simulink model "DC_DC_buck_Microgrid_sim_1_2_3"  (R2023a)
settings: Solver=ode23tb  StartTime=0.0  StopTime=0.05  MaxStep=1/fpwm/200  RelTol=1e-3  EnableMultiTasking=on
values from neighbouring files (symbols this model uses):
  Cf = 2*IoAVmin/(8*fpwm*DeltaVo*Vo)    (= 5.42534722222e-05)    [DC_DC_buck_Microgrid_1_2_3.m]    (also in DC_DC_buck_Microgrid_4.m = 2.71267361111e-05)
  deltaN = Vo/U    (= 0.48)    [DC_DC_buck_Microgrid_1_2_3.m]    (also in DC_DC_buck_Microgrid_4.m)
  fpwm = 10000    [DC_DC_buck_Microgrid_1_2_3.m]    (also in DC_DC_buck_Microgrid_4.m = 20000)
  IoAVmin = Pomin/Vo    (= 2.08333333333)    [DC_DC_buck_Microgrid_1_2_3.m]    (also in DC_DC_buck_Microgrid_4.m)
  Ios = (Pom-Pp-Pomin-Vo^2/Reqp)/Vo    [DC_DC_buck_Microgrid_1_2_3.m]    (also in DC_DC_buck_Microgrid_4.m = 15.625)
  Ki = 1/Tp    (= 153.646401213)    [DC_DC_buck_Microgrid_1_2_3.m]    (also in DC_DC_buck_Microgrid_4.m = 307.292802426)
  Kiv = 1/Tpv    (= 2252.73933103)    [DC_DC_buck_Microgrid_1_2_3.m]    (also in DC_DC_buck_Microgrid_4.m = 4505.47866205)
  Kp = Tz/Tp    (= 0.0678081650224)    [DC_DC_buck_Microgrid_1_2_3.m]    (also in DC_DC_buck_Microgrid_4.m)
  Kpv = Tzv/Tpv    (= 0.187728277586)    [DC_DC_buck_Microgrid_1_2_3.m]    (also in DC_DC_buck_Microgrid_4.m)
  Lf = 1.01*Vo*(1-deltamin)/(2*IoAVmin*fpwm)    (= 0.000677876869565)    [DC_DC_buck_Microgrid_1_2_3.m]    (also in DC_DC_buck_Microgrid_4.m = 0.000338938434783)
  Po = 1500    [DC_DC_buck_Microgrid_1_2_3.m]    (also in DC_DC_buck_Microgrid_4.m)
  Pomin = 100    [DC_DC_buck_Microgrid_1_2_3.m]    (also in DC_DC_buck_Microgrid_4.m)
  ri = 0.01    [DC_DC_buck_Microgrid_1_2_3.m]    (also in DC_DC_buck_Microgrid_4.m)
  Rmax = Vo^2/Pomin    (= 23.04)    [DC_DC_buck_Microgrid_1_2_3.m]    (also in DC_DC_buck_Microgrid_4.m)
  U = 100    [DC_DC_buck_Microgrid_1_2_3.m]    (also in DC_DC_buck_Microgrid_4.m)
  ucmax = 1    [DC_DC_buck_Microgrid_1_2_3.m]    (also in DC_DC_buck_Microgrid_4.m)
  Vo = 48    [DC_DC_buck_Microgrid_1_2_3.m]    (also in DC_DC_buck_Microgrid_4.m)
undefined symbols (not defined in the file or in its folder): Pp
libraries: spsSeriesRLCBranchLib x7, simulink x4, spsCurrentMeasurementLib x3, spsMeanLib x3, spsVoltageMeasurementLib x3, spsControlledCurrentSourceLib x2, spsBreakerLib x1, spsDiodeLib x1, spsIdealSwitchLib x1, spsPWMGeneratorDCDCLib x1, spsMosfetLib x1, spsDCVoltageSourceLib x1
settings Model: Creator=fern  LastModifiedBy=LAFR
settings SolverCC: AlgebraicLoopSolver=TrustRegion
settings DataIOCC: LimitDataPoints=on  SaveFormat=Array  ReturnWorkspaceOutputs=off
settings OptimizationCC: LifeSpan=inf
settings DebuggingCC: UnconnectedInputMsg=warning  UnconnectedOutputMsg=warning  UnconnectedLineMsg=warning  SFUnexpectedBacktrackingDiag=warning  SFNoUnconditionalDefaultTransitionDiag=warning  SFExecutionAtInitializationDiag=none  ArithmeticOperatorsInVariantConditions=warning
settings HardwareCC: ProdBitPerPointer=32  ProdBitPerSizeT=32  ProdBitPerPtrDiffT=32  ProdLargestAtomicFloat=None  ProdIntDivRoundTo=Undefined  ProdEndianess=Unspecified  ProdWordSize=32  ProdHWDeviceType=32-bit Generic
settings ModelReferenceCC: PropagateSignalLabelsOutOfModel=off
settings SFSimCC: SimUseLocalCustomCode=off  CustomCodeUndefinedFunction=UseInterfaceOnly
settings RTWCC: RTWUseLocalCustomCode=off
settings CodeAppCC: StateflowObjectComments=on
settings GRTTargetCC: TargetLangStandard=C89/C90 (ANSI)
settings ConfigComp: CovMetricSettings=dw  CovSaveCumulativeToWorkspaceVar=on  CovSaveSingleToWorkspaceVar=on  CovExternalEMLEnable=off
settings SimscapeCC: SimscapeNormalizeSystem=off

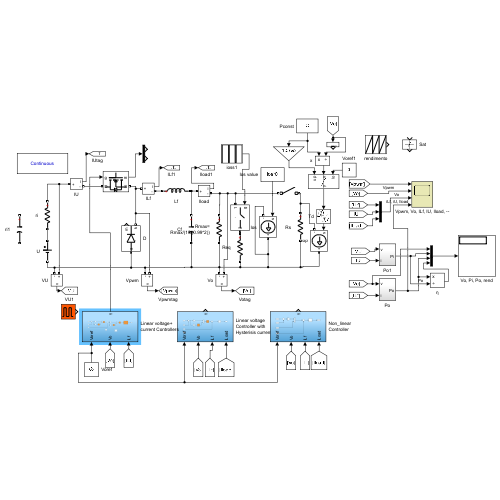
[thumbnail: Simulink's stored preview of the top-level diagram]
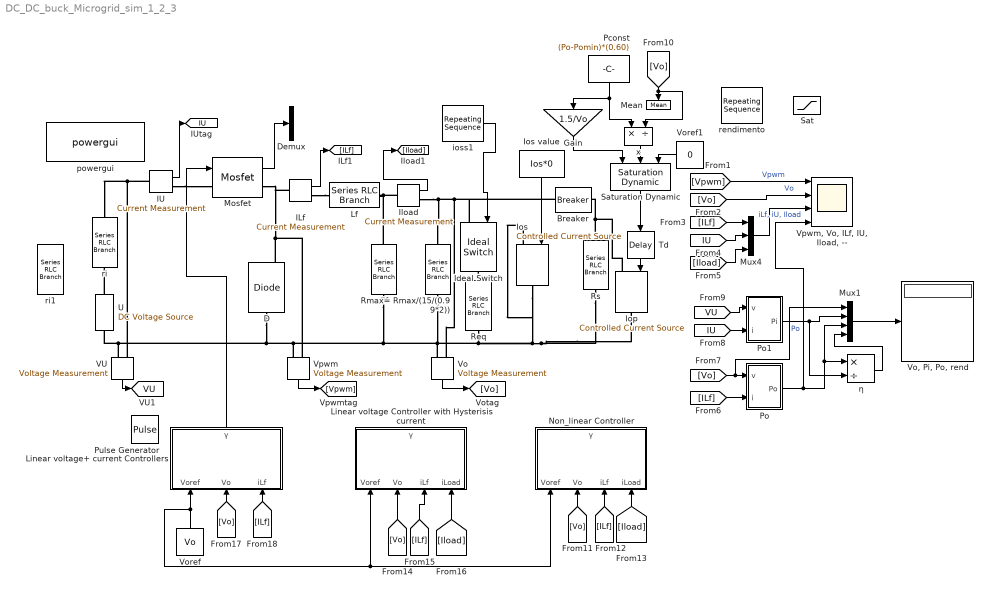
== system DC_DC_buck_Microgrid_sim_1_2_3 ==
  Breaker : spsBreakerLib/Breaker  InitialState=0  SwitchingTimes=[0.02]  External=off  BreakerResistance=0.01  SnubberResistance=Rs  SnubberCapacitance=Cs  Measurements=None  MoreParameters=on  NoBreakLoop=off
  Cf : spsSeriesRLCBranchLib/Series RLC Branch  LConnTagsString=__new0  RConnTagsString=__new0  BranchType=C  Resistance=ri  Inductance=Lf  SetiL0=on  InitialCurrent=IoAVmin  Capacitance=Cf  Setx0=on  InitialVoltage=Vo  Measurements=None
  D : spsDiodeLib/Diode  Ron=Ron  Lon=0  Vf=Vd  IC=0  UseSnubber=off  Rs=Rs  Cs=Cs  Measurements=on
  Demux : Demux  Outputs=2
  Gain : Gain  Gain=1.5/Vo
  ILf : spsCurrentMeasurementLib/Current Measurement  PhasorSimulation=off  OutputType=Complex  PSBequivalent=0
  IU : spsCurrentMeasurementLib/Current Measurement  PhasorSimulation=off  OutputType=Complex  PSBequivalent=0
  Ideal Switch : spsIdealSwitchLib/Ideal Switch  Ron=0.01  Lon=0  IC=0  Rs=Rs  Cs=Cs  Measurements=off
  Iload : spsCurrentMeasurementLib/Current Measurement  PhasorSimulation=off  OutputType=Complex  PSBequivalent=0
  Iop : spsControlledCurrentSourceLib/Controlled Current Source  Initialize=on  Source_Type=DC  Amplitude=0  Phase=0  Frequency=0  Measurements=None
  Ios : spsControlledCurrentSourceLib/Controlled Current Source  Initialize=on  Source_Type=DC  Amplitude=0  Phase=0  Frequency=0  Measurements=None
  Ios value : Constant  Value=Ios*0
  Lf : spsSeriesRLCBranchLib/Series RLC Branch  LConnTagsString=__new0  RConnTagsString=__new0  BranchType=L  Resistance=ri  Inductance=Lf  SetiL0=on  InitialCurrent=IoAVmin  Capacitance=[]  Setx0=off  InitialVoltage=0  Measurements=None
  Linear voltage Controller with Hysterisis current : Subsystem
  Linear voltage+ current Controllers : Subsystem
  Mean : spsMeanLib/Mean  Freq=fpwm/10  Vinit=100  Ts=0
  Mosfet : spsMosfetLib/Mosfet  Ron=Rdson  Lon=0  Rd=Rdson  Vfd=0  IC=0  Rs=Rs  Cs=Cs  Measurements=on
  Mux1 : Mux
  Mux4 : Mux  Inputs=3
  Non_linear Controller : Subsystem
  Pconst : Constant  Value=(Po-Pomin)*(0.60)
  Po : Subsystem
  Po1 : Subsystem
  Pulse Generator : DiscretePulseGenerator  PulseType=Time based  Period=1/fpwm  PulseWidth=deltaN*100
  Req : spsSeriesRLCBranchLib/Series RLC Branch  LConnTagsString=__new0  RConnTagsString=__new0  BranchType=R  Resistance=Vo^2/((Po-Pomin)*(1-0.60))  Inductance=500e-3  SetiL0=on  InitialCurrent=43  Capacitance=[]  Setx0=off  InitialVoltage=0  Measurements=None
  Rmax= Rmax/(15/(0.99*2)) : spsSeriesRLCBranchLib/Series RLC Branch  LConnTagsString=__new0  RConnTagsString=__new0  BranchType=R  Resistance=Rmax  Inductance=500e-3  SetiL0=on  InitialCurrent=43  Capacitance=[]  Setx0=off  InitialVoltage=0  Measurements=None
  Rs : spsSeriesRLCBranchLib/Series RLC Branch  LConnTagsString=__new0  RConnTagsString=__new0  BranchType=R  Resistance=1000*Rmax  Inductance=500e-3  SetiL0=on  InitialCurrent=43  Capacitance=[]  Setx0=off  InitialVoltage=0  Measurements=None
  Sat : Saturate  UpperLimit=Pp*1.5/Vo  LowerLimit=0
  Saturation Dynamic : simulink/Discontinuities/Saturation Dynamic  OutMin=[]  OutMax=[]  OutDataTypeStr=Inherit: Same as second input  OutDataType=fixdt(1, 16)  OutScaling=2^-10  DoSatur=off
  Td : TransportDelay  DelayTime=1/(2*fpwm)  BufferSize=2048
  U : spsDCVoltageSourceLib/DC Voltage Source  Description=source block  Amplitude=U  Measurements=None
      settings: AttributesFormatString=\n
  VU : spsVoltageMeasurementLib/Voltage Measurement  Tag=PoWeRsYsTeMmEaSuReMeNt  PhasorSimulation=off  OutputType=Complex  PSBequivalent=0
  Vo : spsVoltageMeasurementLib/Voltage Measurement  Tag=PoWeRsYsTeMmEaSuReMeNt  PhasorSimulation=off  OutputType=Complex  PSBequivalent=0
  "Vo, Pi, Po, rend" : Display
      settings: Decimation=1000
  Voref : Constant  Value=Vo
  Voref1 : Constant  Value=0
  Vpwm : spsVoltageMeasurementLib/Voltage Measurement  Tag=PoWeRsYsTeMmEaSuReMeNt  PhasorSimulation=off  OutputType=Complex  PSBequivalent=0
  "Vpwm, Vo, ILf, IU, Iload, --" : Scope  NumInputPorts=4
  ioss1 : simulink/Sources/Repeating Sequence  rep_seq_t=[0 0.009 0.01 0.1]  rep_seq_y=[0 0 1 1 ]
  powergui : spspowerguiLib/powergui  Priority=2  SimulationMode=Continuous  SampleTime=0  frequency=60  Iterations=50  frequencyindice=0  Pbase=100e6  ErrMax=1e-4  UnitsV=kV  UnitsW=MW  buscounter=0  FunctionMessages=off  echomessages=off  EnableUseOfTLC=off  CurrentSourceSwitches=on  DisableSnubberDevices=off  DisableRonSwitches=off  DisableVfSwitches=off  DisplayEquations=off  AutomaticDiscreteSolvers=off  SolverType=Tustin/Backward Euler (TBE)  Interpol=off  ExternalGateDelay=off  methode=off  Ts=0  x0status=blocks  SPID=off  SwTol=0  HookPort=off  NonlinearTolerance=1e-4  nMaxIteration=100  ContinueOnMaxIteration=off  RestoreLinks=warning  ResistiveCurrentMeasurement=off  Frange=[0:2:500]  Ylog=off  Xlog=on  ShowGrid=off  save=off  variable=ZData  structure=psbconverter_str  ZoomFFT=on  StartTime=0.1-2/60  cycles=2  DisplayStyle=off  fundamental=60  FreqAxis=on  MaxFrequency=2000  frequencyindicesteady=1  RmsSteady=1  display=off
  rendimento : simulink/Sources/Repeating Sequence  rep_seq_t=[0 0.1]  rep_seq_y=[0 30]
  ri : spsSeriesRLCBranchLib/Series RLC Branch  LConnTagsString=__new0  RConnTagsString=__new0  BranchType=R  Resistance=ri  Inductance=1e-6  SetiL0=off  InitialCurrent=4  Capacitance=[]  Setx0=off  InitialVoltage=0  Measurements=None
  ri1 : spsSeriesRLCBranchLib/Series RLC Branch  LConnTagsString=__new0  RConnTagsString=__new0  BranchType=C  Resistance=ri  Inductance=1e-6  SetiL0=off  InitialCurrent=4  Capacitance=100e-6  Setx0=on  InitialVoltage=U  Measurements=None
  x : Product  Inputs=*/
  η : Product  Inputs=*/
  tag scope: IU=global, VU=global
  wires:
  Pconst/1 -> Gain/1, x/1
  Vo/1 -> [Vo]
  [Vpwm] -> "Vpwm, Vo, ILf, IU, Iload, --"/1  "Vpwm"
  [Vo] -> "Vpwm, Vo, ILf, IU, Iload, --"/2  "Vo"
  Iload/1 -> [Iload]
  ILf/1 -> [ILf]
  [ILf] -> Mux4/1
  [IU] -> Mux4/2
  [Iload] -> Mux4/3
  Mux4/1 -> "Vpwm, Vo, ILf, IU, Iload, --"/3  "iLf, iU, Iload"
  [Vo] -> Mux1/1, Po/1(v)
  [ILf] -> Po/2(i)
  Po/1(Po) -> "Vpwm, Vo, ILf, IU, Iload, --"/4, Mux1/3, η/1  "Po"
  Mux1/1 -> "Vo, Pi, Po, rend"/1
  VU/1 -> [VU]
  Vpwm/1 -> [Vpwm]
  [VU] -> Po1/1(v)
  [IU] -> Po1/2(i)
  Mosfet/1 -> Demux/1
  IU/1 -> [IU]
  Po1/1(Pi) -> η/2, Mux1/2
  η/1 -> Mux1/4
  x/1 -> Saturation Dynamic/2
  [Iload] -> Linear voltage Controller with Hysterisis current/4(iLoad)
  [ILf] -> Linear voltage Controller with Hysterisis current/3(iLf)
  [Vo] -> Linear voltage Controller with Hysterisis current/2(Vo)
  Voref/1 -> Linear voltage+ current Controllers/1(Voref), Non_linear Controller/1(Voref), Linear voltage Controller with Hysterisis current/1(Voref)
  [Vo] -> Non_linear Controller/2(Vo)
  [ILf] -> Non_linear Controller/3(iLf)
  [Iload] -> Non_linear Controller/4(iLoad)
  [ILf] -> Linear voltage+ current Controllers/3(iLf)
  [Vo] -> Linear voltage+ current Controllers/2(Vo)
  Td/1 -> Iop/1
  Ios value/1 -> Ios/1
  ioss1/1 -> Ideal Switch/1
  [Vo] -> Mean/1, x/2
  Linear voltage+ current Controllers/1(γ) -> Mosfet/1
  Saturation Dynamic/1 -> Td/1
  Voref1/1 -> Saturation Dynamic/3
  Gain/1 -> Saturation Dynamic/1
  connections:
  U/RConn1 -- ri/RConn1
  VU/LConn1 -- IU/LConn1 -- ri/LConn1
  D/RConn1 -- Mosfet/RConn1 -- ILf/LConn1 -- Vpwm/LConn1
  D/LConn1 -- Req/RConn1 -- Ios/LConn1 -- Ios/RConn1 -- Rs/RConn1 -- Iop/RConn1 -- Rmax= Rmax/(15/(0.99*2))/RConn1 -- Vo/LConn2 -- Cf/RConn1 -- Vpwm/LConn2 -- VU/LConn2 -- U/LConn1
  Iload/RConn1 -- Ideal Switch/LConn1 -- Breaker/LConn1 -- Vo/LConn1 -- Rmax= Rmax/(15/(0.99*2))/LConn1
  Cf/LConn1 -- Lf/RConn1 -- Iload/LConn1
  ILf/RConn1 -- Lf/LConn1
  IU/RConn1 -- Mosfet/LConn1
  Rs/LConn1 -- Iop/LConn1 -- Breaker/RConn1
  Req/LConn1 -- Ideal Switch/RConn1

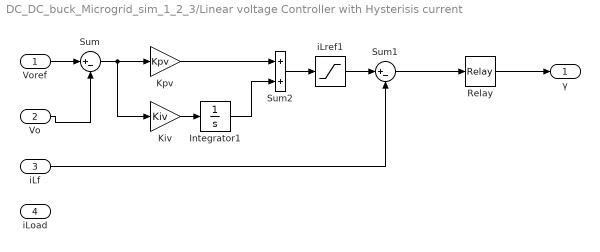
== system DC_DC_buck_Microgrid_sim_1_2_3/Linear voltage Controller with Hysterisis current ==
  Voref : Inport
  Vo : Inport  Port=2
  iLf : Inport  Port=3
  iLoad : Inport  Port=4
  Integrator1 : Integrator  LimitOutput=on  UpperSaturationLimit=60  LowerSaturationLimit=-60
  Kiv : Gain  Gain=Kiv
  Kpv : Gain  Gain=Kpv
  Relay : Relay  OnSwitchValue=IoAVmin/2  OffSwitchValue=-IoAVmin/2
  Sum : Sum  Inputs=|+-
  Sum1 : Sum  Inputs=|+-
  Sum2 : Sum
  iLref1 : Saturate  UpperLimit=60  LowerLimit=0
  γ : Outport
  wires:
  Kpv/1 -> Sum2/1
  Sum1/1 -> Relay/1
  Sum/1 -> Kiv/1, Kpv/1
  Vo/1 -> Sum/2
  Voref/1 -> Sum/1
  Relay/1 -> γ/1
  Sum2/1 -> iLref1/1
  iLf/1 -> Sum1/2
  Kiv/1 -> Integrator1/1
  Integrator1/1 -> Sum2/2
  iLref1/1 -> Sum1/1

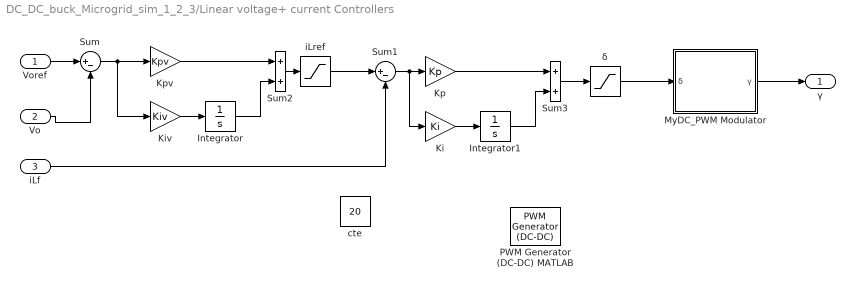
== system DC_DC_buck_Microgrid_sim_1_2_3/Linear voltage+ current Controllers ==
  Voref : Inport
  Vo : Inport  Port=2
  iLf : Inport  Port=3
  Integrator : Integrator  LimitOutput=on  UpperSaturationLimit=1  LowerSaturationLimit=-1
  Integrator1 : Integrator  LimitOutput=on  UpperSaturationLimit=1  LowerSaturationLimit=-1
  Ki : Gain  Gain=Ki
  Kiv : Gain  Gain=Kiv
  Kp : Gain  Gain=Kp
  Kpv : Gain  Gain=Kpv
  MyDC_PWM Modulator : Subsystem
  PWM Generator (DC-DC) MATLAB : spsPWMGeneratorDCDCLib/PWM Generator (DC-DC)  Fsw=fpwm  Ts=0
  Sum : Sum  Inputs=|+-
  Sum1 : Sum  Inputs=|+-
  Sum2 : Sum
  Sum3 : Sum
  cte : Constant  Value=20
  iLref : Saturate  UpperLimit=60  LowerLimit=0
  δ : Saturate  UpperLimit=0.99  LowerLimit=0.01
  γ : Outport
  wires:
  Integrator/1 -> Sum2/2
  Kiv/1 -> Integrator/1
  iLf/1 -> Sum1/2
  Sum2/1 -> iLref/1
  Voref/1 -> Sum/1
  Vo/1 -> Sum/2
  Sum/1 -> Kpv/1, Kiv/1
  Kpv/1 -> Sum2/1
  Integrator1/1 -> Sum3/2
  Ki/1 -> Integrator1/1
  Sum3/1 -> δ/1
  Sum1/1 -> Kp/1, Ki/1
  Kp/1 -> Sum3/1
  iLref/1 -> Sum1/1
  δ/1 -> MyDC_PWM Modulator/1(δ)
  MyDC_PWM Modulator/1(γ) -> γ/1

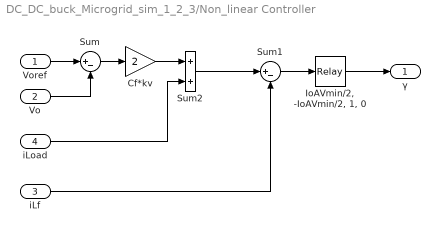
== system DC_DC_buck_Microgrid_sim_1_2_3/Non_linear Controller ==
  Voref : Inport
  Vo : Inport  Port=2
  iLf : Inport  Port=3
  iLoad : Inport  Port=4
  Cf*kv : Gain  Gain=2
  "IoAVmin/2, -IoAVmin/2, 1, 0" : Relay  OnSwitchValue=IoAVmin/2  OffSwitchValue=-IoAVmin/2
  Sum : Sum  Inputs=|+-
  Sum1 : Sum  Inputs=|+-
  Sum2 : Sum
  γ : Outport
  wires:
  "IoAVmin/2, -IoAVmin/2, 1, 0"/1 -> γ/1
  Voref/1 -> Sum/1
  Vo/1 -> Sum/2
  Sum/1 -> Cf*kv/1
  iLf/1 -> Sum1/2
  Sum1/1 -> "IoAVmin/2, -IoAVmin/2, 1, 0"/1
  Cf*kv/1 -> Sum2/1
  Sum2/1 -> Sum1/1
  iLoad/1 -> Sum2/2

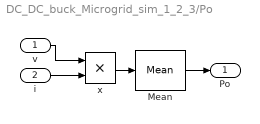
== system DC_DC_buck_Microgrid_sim_1_2_3/Po ==
  v : Inport
  i : Inport  Port=2
  Mean : spsMeanLib/Mean  Freq=fpwm/10  Vinit=100  Ts=0
  x : Product  Inputs=**
  Po : Outport
  wires:
  x/1 -> Mean/1
  v/1 -> x/1
  i/1 -> x/2
  Mean/1 -> Po/1

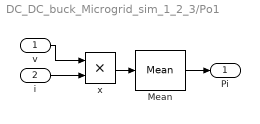
== system DC_DC_buck_Microgrid_sim_1_2_3/Po1 ==
  v : Inport
  i : Inport  Port=2
  Mean : spsMeanLib/Mean  Freq=fpwm/10  Vinit=110  Ts=0
  x : Product  Inputs=**
  Pi : Outport
  wires:
  Mean/1 -> Pi/1
  i/1 -> x/2
  v/1 -> x/1
  x/1 -> Mean/1

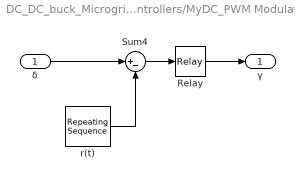
== system DC_DC_buck_Microgrid_sim_1_2_3/Linear voltage+ current Controllers/MyDC_PWM Modulator ==
  δ : Inport
  Relay : Relay  OnSwitchValue=0.01  OffSwitchValue=-0.01
  Sum4 : Sum  Inputs=|+-
  r(t) : simulink/Sources/Repeating Sequence  rep_seq_t=[0 1/fpwm]  rep_seq_y=[0 ucmax]
  γ : Outport
  wires:
  Relay/1 -> γ/1
  r(t)/1 -> Sum4/2
  Sum4/1 -> Relay/1
  δ/1 -> Sum4/1
